simulink model "inverter_model"  (R2018b)
settings: Solver=VariableStepAuto  StartTime=0.0  StopTime=0.75  MaxStep=0.01  RelTol=1e-3  EnableMultiTasking=on
undefined symbols (not defined in the file): L, Lf, R, ron
libraries: powerlib x46, powerlib_meascontrol x11, simulink x9, peTransforms x5, simulink_extras x1
settings Model: Creator=vm-user  LastModifiedBy=suku (WPC)
settings DataIOCC: LimitDataPoints=on  SaveOutput=off  SaveTime=off
settings OptimizationCC: ExpressionDepthLimit=2147483647  LifeSpan=1
settings DebuggingCC: UnderspecifiedInitializationDetection=Classic  MergeDetectMultiDrivingBlocksExec=none  FcnCallInpInsideContextMsg=warning  AllowSymbolicDim=off  StateNameClashWarn=warning  LibraryContextMissingDiagnostic=none  SFUnexpectedBacktrackingDiag=warning  SFNoUnconditionalDefaultTransitionDiag=warning  SFExecutionAtInitializationDiag=none
settings SFSimCC: SimUseLocalCustomCode=off
settings RTWCC: RTWUseLocalCustomCode=off
settings CodeAppCC: StateflowObjectComments=on
settings GRTTargetCC: TargetLangStandard=C89/C90 (ANSI)  GeneratePreprocessorConditionals=Disable all  CombineOutputUpdateFcns=off  GRTInterface=on

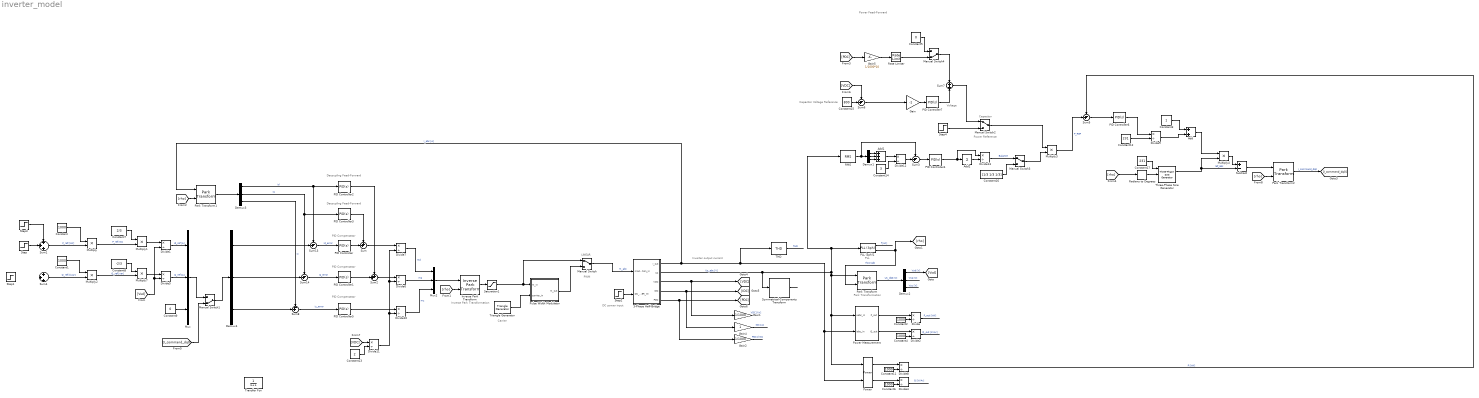
== system inverter_model ==
  note: Power Reference
  note: PLL
  note: PID Compensator
  note: PWM
  note: LINEAR
  note: Carrier
  note: Park Transformation
  note: Inverse Park Transformation
  note: Inverter output current
  note: Decoupling Feed-Forward
  note: Decoupling Feed-Forward
  note: Capacitor
  note: Capacitor Voltage Reference
  note: Power Feed-Forward
  note: Voltage
  note: DC power input
  note: PID Compensator
  note: PID Compensator
  3-Phase Half-Bridge : Subsystem
  Add : Sum
  Add1 : Sum  Inputs=+++
  Add2 : Sum  Inputs=+
  Constant{,1..2,4,6,11} (6 alike) : Constant  Value=1000
  Constant12 : Constant  Value=231
  Constant13 : Constant  Value=2
  Constant14 : Constant  Value=3
  Constant15 : Constant  Value=800
  Constant16 : Constant  Value=[1/3 1/3 1/3]
  Constant17 : Constant  Value=231
  Constant3 : Constant
  Constant5 : Constant  Value=0
  Constant7 : Constant  Value=2/3
  Constant8 : Constant  Value=-2/3
  Constant9 : Constant  Value=0
  Demux{1..4} (4 alike) : Demux  Outputs=3
  Divide{,1..2,4..13} (13 alike) : Product  Inputs=*/
  Gain : Gain  Gain=-1
  Gain1 : Gain  Gain=1/1000
  Gain2 : Gain  Gain=1/1000
  Gain4 : Gain
  Gain5 : Gain  Gain=1/1000*10
  Inverse Park Transform : peTransforms/Inverse Park Transform  AxisAlignment=Q-axis  PowerInvariant=off
  Manual Switch : ManualSwitch
  Manual Switch1 : ManualSwitch  CurrentSetting=0
  Manual Switch2 : ManualSwitch
  Manual Switch3 : ManualSwitch
  Manual Switch4 : ManualSwitch  CurrentSetting=0
  Multiply{,1..4,7} (6 alike) : Product
  Mux : Mux  Inputs=3
  Mux2 : Mux  Inputs=3
  PID Controller : simulink/Continuous/PID Controller  Controller=PID  Form=Parallel  TimeDomain=Continuous-time  SampleTime=-1  IntegratorMethod=Forward Euler  FilterMethod=Forward Euler  ControllerParametersSource=internal  P=1  I=100  D=0.25  UseFilter=on  N=100  TunerSelectOption=Transfer Function Based (PID Tuner App)  InitialConditionSource=internal  InitialConditionForIntegrator=0  InitialConditionForFilter=0  DifferentiatorICPrevScaledInput=0  ExternalReset=none  TrackingMode=off  Kt=1  LimitOutput=off  UpperSaturationLimit=inf  LowerSaturationLimit=-inf  LinearizeAsGain=on  AntiWindupMode=none  Kb=1  POutMin=[]  POutMax=[]  IOutMin=[]  IOutMax=[]  DOutMin=[]  DOutMax=[]  NOutMin=[]  NOutMax=[]  SumOutMin=[]  SumOutMax=[]  SaturationOutMin=[]  SaturationOutMax=[]  PParamMin=[]  PParamMax=[]  IParamMin=[]  IParamMax=[]  DParamMin=[]  DParamMax=[]  NParamMin=[]  NParamMax=[]  KbParamMin=[]  KbParamMax=[]  KtParamMin=[]  KtParamMax=[]  KbOutMin=[]  KbOutMax=[]  KtOutMin=[]  KtOutMax=[]  IntegratorOutMin=[]  IntegratorOutMax=[]  FilterOutMin=[]  FilterOutMax=[]  SumI1OutMin=[]  SumI1OutMax=[]  SumI2OutMin=[]  SumI2OutMax=[]  SumI3OutMin=[]  SumI3OutMax=[]  SumI4OutMin=[]  SumI4OutMax=[]  SumDOutMin=[]  SumDOutMax=[]  DifferentiatorOutMin=[]  DifferentiatorOutMax=[]  FilterDiffOutCoefMin=[]  FilterDiffOutCoefMax=[]  ReciprocalOutMin=[]  ReciprocalOutMax=[]  SumDenOutMin=[]  SumDenOutMax=[]  SumNumOutMin=[]  SumNumOutMax=[]  DivideOutMin=[]  DivideOutMax=[]  IntegratorContinuousStateAttributes=''  IntegratorStateMustResolveToSignalObject=off  IntegratorRTWStateStorageClass=Auto  FilterContinuousStateAttributes=''  FilterStateMustResolveToSignalObject=off  FilterRTWStateStorageClass=Auto  ParallelPVariant=InternalParameters  IdealPVariant=Disabled  IVariant=InternalParameters  DVariant=InternalParameters  IntegratorVariant=Continuous  SatVariant=Disabled  AWVariant=Passthrough  PCopyVariant=Disabled  TRVariant=Disabled  FdbkBlocksVariant=Forward  IdealPFdbkVariant=Disabled  SatFdbkVariant=Disabled  DerivativeFilterVariant=ContFilter  NVariant=InternalParameters  NCopyVariant=Disabled  FilterICVariant=InternalICsFilter  IntegratorICVariant=InternalICs  ExternalResetVariant=Disabled  TRSumVariant=Passthrough  SumFdbkVariant=Disabled  SumVariant=Sum_PID
  PID Controller1 : simulink/Continuous/PID Controller  Controller=PID  Form=Parallel  TimeDomain=Continuous-time  SampleTime=-1  IntegratorMethod=Forward Euler  FilterMethod=Forward Euler  ControllerParametersSource=internal  P=1  I=100  D=0.25  UseFilter=on  N=100  TunerSelectOption=Transfer Function Based (PID Tuner App)  InitialConditionSource=internal  InitialConditionForIntegrator=0  InitialConditionForFilter=0  DifferentiatorICPrevScaledInput=0  ExternalReset=none  TrackingMode=off  Kt=1  LimitOutput=off  UpperSaturationLimit=inf  LowerSaturationLimit=-inf  LinearizeAsGain=on  AntiWindupMode=none  Kb=1  POutMin=[]  POutMax=[]  IOutMin=[]  IOutMax=[]  DOutMin=[]  DOutMax=[]  NOutMin=[]  NOutMax=[]  SumOutMin=[]  SumOutMax=[]  SaturationOutMin=[]  SaturationOutMax=[]  PParamMin=[]  PParamMax=[]  IParamMin=[]  IParamMax=[]  DParamMin=[]  DParamMax=[]  NParamMin=[]  NParamMax=[]  KbParamMin=[]  KbParamMax=[]  KtParamMin=[]  KtParamMax=[]  KbOutMin=[]  KbOutMax=[]  KtOutMin=[]  KtOutMax=[]  IntegratorOutMin=[]  IntegratorOutMax=[]  FilterOutMin=[]  FilterOutMax=[]  SumI1OutMin=[]  SumI1OutMax=[]  SumI2OutMin=[]  SumI2OutMax=[]  SumI3OutMin=[]  SumI3OutMax=[]  SumI4OutMin=[]  SumI4OutMax=[]  SumDOutMin=[]  SumDOutMax=[]  DifferentiatorOutMin=[]  DifferentiatorOutMax=[]  FilterDiffOutCoefMin=[]  FilterDiffOutCoefMax=[]  ReciprocalOutMin=[]  ReciprocalOutMax=[]  SumDenOutMin=[]  SumDenOutMax=[]  SumNumOutMin=[]  SumNumOutMax=[]  DivideOutMin=[]  DivideOutMax=[]  IntegratorContinuousStateAttributes=''  IntegratorStateMustResolveToSignalObject=off  IntegratorRTWStateStorageClass=Auto  FilterContinuousStateAttributes=''  FilterStateMustResolveToSignalObject=off  FilterRTWStateStorageClass=Auto  ParallelPVariant=InternalParameters  IdealPVariant=Disabled  IVariant=InternalParameters  DVariant=InternalParameters  IntegratorVariant=Continuous  SatVariant=Disabled  AWVariant=Passthrough  PCopyVariant=Disabled  TRVariant=Disabled  FdbkBlocksVariant=Forward  IdealPFdbkVariant=Disabled  SatFdbkVariant=Disabled  DerivativeFilterVariant=ContFilter  NVariant=InternalParameters  NCopyVariant=Disabled  FilterICVariant=InternalICsFilter  IntegratorICVariant=InternalICs  ExternalResetVariant=Disabled  TRSumVariant=Passthrough  SumFdbkVariant=Disabled  SumVariant=Sum_PID
  PID Controller2 : simulink/Continuous/PID Controller  Controller=PID  Form=Parallel  TimeDomain=Continuous-time  SampleTime=-1  IntegratorMethod=Forward Euler  FilterMethod=Forward Euler  ControllerParametersSource=internal  P=0.22  I=0  D=0  UseFilter=on  N=100  TunerSelectOption=Transfer Function Based (PID Tuner App)  InitialConditionSource=internal  InitialConditionForIntegrator=0  InitialConditionForFilter=0  DifferentiatorICPrevScaledInput=0  ExternalReset=none  TrackingMode=off  Kt=1  LimitOutput=off  UpperSaturationLimit=inf  LowerSaturationLimit=-inf  LinearizeAsGain=on  AntiWindupMode=none  Kb=1  POutMin=[]  POutMax=[]  IOutMin=[]  IOutMax=[]  DOutMin=[]  DOutMax=[]  NOutMin=[]  NOutMax=[]  SumOutMin=[]  SumOutMax=[]  SaturationOutMin=[]  SaturationOutMax=[]  PParamMin=[]  PParamMax=[]  IParamMin=[]  IParamMax=[]  DParamMin=[]  DParamMax=[]  NParamMin=[]  NParamMax=[]  KbParamMin=[]  KbParamMax=[]  KtParamMin=[]  KtParamMax=[]  KbOutMin=[]  KbOutMax=[]  KtOutMin=[]  KtOutMax=[]  IntegratorOutMin=[]  IntegratorOutMax=[]  FilterOutMin=[]  FilterOutMax=[]  SumI1OutMin=[]  SumI1OutMax=[]  SumI2OutMin=[]  SumI2OutMax=[]  SumI3OutMin=[]  SumI3OutMax=[]  SumI4OutMin=[]  SumI4OutMax=[]  SumDOutMin=[]  SumDOutMax=[]  DifferentiatorOutMin=[]  DifferentiatorOutMax=[]  FilterDiffOutCoefMin=[]  FilterDiffOutCoefMax=[]  ReciprocalOutMin=[]  ReciprocalOutMax=[]  SumDenOutMin=[]  SumDenOutMax=[]  SumNumOutMin=[]  SumNumOutMax=[]  DivideOutMin=[]  DivideOutMax=[]  IntegratorContinuousStateAttributes=''  IntegratorStateMustResolveToSignalObject=off  IntegratorRTWStateStorageClass=Auto  FilterContinuousStateAttributes=''  FilterStateMustResolveToSignalObject=off  FilterRTWStateStorageClass=Auto  ParallelPVariant=InternalParameters  IdealPVariant=Disabled  IVariant=InternalParameters  DVariant=InternalParameters  IntegratorVariant=Continuous  SatVariant=Disabled  AWVariant=Passthrough  PCopyVariant=Disabled  TRVariant=Disabled  FdbkBlocksVariant=Forward  IdealPFdbkVariant=Disabled  SatFdbkVariant=Disabled  DerivativeFilterVariant=ContFilter  NVariant=InternalParameters  NCopyVariant=Disabled  FilterICVariant=InternalICsFilter  IntegratorICVariant=InternalICs  ExternalResetVariant=Disabled  TRSumVariant=Passthrough  SumFdbkVariant=Disabled  SumVariant=Sum_PID
  PID Controller3 : simulink/Continuous/PID Controller  Controller=PID  Form=Parallel  TimeDomain=Continuous-time  SampleTime=-1  IntegratorMethod=Forward Euler  FilterMethod=Forward Euler  ControllerParametersSource=internal  P=-0.22  I=0  D=0  UseFilter=on  N=100  TunerSelectOption=Transfer Function Based (PID Tuner App)  InitialConditionSource=internal  InitialConditionForIntegrator=0  InitialConditionForFilter=0  DifferentiatorICPrevScaledInput=0  ExternalReset=none  TrackingMode=off  Kt=1  LimitOutput=off  UpperSaturationLimit=inf  LowerSaturationLimit=-inf  LinearizeAsGain=on  AntiWindupMode=none  Kb=1  POutMin=[]  POutMax=[]  IOutMin=[]  IOutMax=[]  DOutMin=[]  DOutMax=[]  NOutMin=[]  NOutMax=[]  SumOutMin=[]  SumOutMax=[]  SaturationOutMin=[]  SaturationOutMax=[]  PParamMin=[]  PParamMax=[]  IParamMin=[]  IParamMax=[]  DParamMin=[]  DParamMax=[]  NParamMin=[]  NParamMax=[]  KbParamMin=[]  KbParamMax=[]  KtParamMin=[]  KtParamMax=[]  KbOutMin=[]  KbOutMax=[]  KtOutMin=[]  KtOutMax=[]  IntegratorOutMin=[]  IntegratorOutMax=[]  FilterOutMin=[]  FilterOutMax=[]  SumI1OutMin=[]  SumI1OutMax=[]  SumI2OutMin=[]  SumI2OutMax=[]  SumI3OutMin=[]  SumI3OutMax=[]  SumI4OutMin=[]  SumI4OutMax=[]  SumDOutMin=[]  SumDOutMax=[]  DifferentiatorOutMin=[]  DifferentiatorOutMax=[]  FilterDiffOutCoefMin=[]  FilterDiffOutCoefMax=[]  ReciprocalOutMin=[]  ReciprocalOutMax=[]  SumDenOutMin=[]  SumDenOutMax=[]  SumNumOutMin=[]  SumNumOutMax=[]  DivideOutMin=[]  DivideOutMax=[]  IntegratorContinuousStateAttributes=''  IntegratorStateMustResolveToSignalObject=off  IntegratorRTWStateStorageClass=Auto  FilterContinuousStateAttributes=''  FilterStateMustResolveToSignalObject=off  FilterRTWStateStorageClass=Auto  ParallelPVariant=InternalParameters  IdealPVariant=Disabled  IVariant=InternalParameters  DVariant=InternalParameters  IntegratorVariant=Continuous  SatVariant=Disabled  AWVariant=Passthrough  PCopyVariant=Disabled  TRVariant=Disabled  FdbkBlocksVariant=Forward  IdealPFdbkVariant=Disabled  SatFdbkVariant=Disabled  DerivativeFilterVariant=ContFilter  NVariant=InternalParameters  NCopyVariant=Disabled  FilterICVariant=InternalICsFilter  IntegratorICVariant=InternalICs  ExternalResetVariant=Disabled  TRSumVariant=Passthrough  SumFdbkVariant=Disabled  SumVariant=Sum_PID
  PID Controller4 : simulink/Continuous/PID Controller  Controller=PID  Form=Parallel  TimeDomain=Continuous-time  SampleTime=-1  IntegratorMethod=Forward Euler  FilterMethod=Forward Euler  ControllerParametersSource=internal  P=0.1  I=1  D=0  UseFilter=on  N=100  TunerSelectOption=Transfer Function Based (PID Tuner App)  InitialConditionSource=internal  InitialConditionForIntegrator=1/3  InitialConditionForFilter=0  DifferentiatorICPrevScaledInput=0  ExternalReset=none  TrackingMode=off  Kt=1  LimitOutput=on  UpperSaturationLimit=0.9  LowerSaturationLimit=0.1  LinearizeAsGain=on  AntiWindupMode=clamping  Kb=1  POutMin=[]  POutMax=[]  IOutMin=[]  IOutMax=[]  DOutMin=[]  DOutMax=[]  NOutMin=[]  NOutMax=[]  SumOutMin=[]  SumOutMax=[]  SaturationOutMin=[]  SaturationOutMax=[]  PParamMin=[]  PParamMax=[]  IParamMin=[]  IParamMax=[]  DParamMin=[]  DParamMax=[]  NParamMin=[]  NParamMax=[]  KbParamMin=[]  KbParamMax=[]  KtParamMin=[]  KtParamMax=[]  KbOutMin=[]  KbOutMax=[]  KtOutMin=[]  KtOutMax=[]  IntegratorOutMin=[]  IntegratorOutMax=[]  FilterOutMin=[]  FilterOutMax=[]  SumI1OutMin=[]  SumI1OutMax=[]  SumI2OutMin=[]  SumI2OutMax=[]  SumI3OutMin=[]  SumI3OutMax=[]  SumI4OutMin=[]  SumI4OutMax=[]  SumDOutMin=[]  SumDOutMax=[]  DifferentiatorOutMin=[]  DifferentiatorOutMax=[]  FilterDiffOutCoefMin=[]  FilterDiffOutCoefMax=[]  ReciprocalOutMin=[]  ReciprocalOutMax=[]  SumDenOutMin=[]  SumDenOutMax=[]  SumNumOutMin=[]  SumNumOutMax=[]  DivideOutMin=[]  DivideOutMax=[]  IntegratorContinuousStateAttributes=''  IntegratorStateMustResolveToSignalObject=off  IntegratorRTWStateStorageClass=Auto  FilterContinuousStateAttributes=''  FilterStateMustResolveToSignalObject=off  FilterRTWStateStorageClass=Auto  ParallelPVariant=InternalParameters  IdealPVariant=Disabled  IVariant=InternalParameters  DVariant=InternalParameters  IntegratorVariant=Continuous  SatVariant=Enabled  AWVariant=ContClampingParallel  PCopyVariant=Disabled  TRVariant=Disabled  FdbkBlocksVariant=Forward  IdealPFdbkVariant=Disabled  SatFdbkVariant=Disabled  DerivativeFilterVariant=ContFilter  NVariant=InternalParameters  NCopyVariant=Disabled  FilterICVariant=InternalICsFilter  IntegratorICVariant=InternalICs  ExternalResetVariant=Disabled  TRSumVariant=Passthrough  SumFdbkVariant=Disabled  SumVariant=Sum_PID
  PID Controller5 : simulink/Continuous/PID Controller  Controller=PID  Form=Parallel  TimeDomain=Continuous-time  SampleTime=-1  IntegratorMethod=Forward Euler  FilterMethod=Forward Euler  ControllerParametersSource=internal  P=1  I=100  D=0.25  UseFilter=on  N=100  TunerSelectOption=Transfer Function Based (PID Tuner App)  InitialConditionSource=internal  InitialConditionForIntegrator=0  InitialConditionForFilter=0  DifferentiatorICPrevScaledInput=0  ExternalReset=none  TrackingMode=off  Kt=1  LimitOutput=off  UpperSaturationLimit=inf  LowerSaturationLimit=-inf  LinearizeAsGain=on  AntiWindupMode=none  Kb=1  POutMin=[]  POutMax=[]  IOutMin=[]  IOutMax=[]  DOutMin=[]  DOutMax=[]  NOutMin=[]  NOutMax=[]  SumOutMin=[]  SumOutMax=[]  SaturationOutMin=[]  SaturationOutMax=[]  PParamMin=[]  PParamMax=[]  IParamMin=[]  IParamMax=[]  DParamMin=[]  DParamMax=[]  NParamMin=[]  NParamMax=[]  KbParamMin=[]  KbParamMax=[]  KtParamMin=[]  KtParamMax=[]  KbOutMin=[]  KbOutMax=[]  KtOutMin=[]  KtOutMax=[]  IntegratorOutMin=[]  IntegratorOutMax=[]  FilterOutMin=[]  FilterOutMax=[]  SumI1OutMin=[]  SumI1OutMax=[]  SumI2OutMin=[]  SumI2OutMax=[]  SumI3OutMin=[]  SumI3OutMax=[]  SumI4OutMin=[]  SumI4OutMax=[]  SumDOutMin=[]  SumDOutMax=[]  DifferentiatorOutMin=[]  DifferentiatorOutMax=[]  FilterDiffOutCoefMin=[]  FilterDiffOutCoefMax=[]  ReciprocalOutMin=[]  ReciprocalOutMax=[]  SumDenOutMin=[]  SumDenOutMax=[]  SumNumOutMin=[]  SumNumOutMax=[]  DivideOutMin=[]  DivideOutMax=[]  IntegratorContinuousStateAttributes=''  IntegratorStateMustResolveToSignalObject=off  IntegratorRTWStateStorageClass=Auto  FilterContinuousStateAttributes=''  FilterStateMustResolveToSignalObject=off  FilterRTWStateStorageClass=Auto  ParallelPVariant=InternalParameters  IdealPVariant=Disabled  IVariant=InternalParameters  DVariant=InternalParameters  IntegratorVariant=Continuous  SatVariant=Disabled  AWVariant=Passthrough  PCopyVariant=Disabled  TRVariant=Disabled  FdbkBlocksVariant=Forward  IdealPFdbkVariant=Disabled  SatFdbkVariant=Disabled  DerivativeFilterVariant=ContFilter  NVariant=InternalParameters  NCopyVariant=Disabled  FilterICVariant=InternalICsFilter  IntegratorICVariant=InternalICs  ExternalResetVariant=Disabled  TRSumVariant=Passthrough  SumFdbkVariant=Disabled  SumVariant=Sum_PID
  PID Controller6 : simulink/Continuous/PID Controller  Controller=PID  Form=Parallel  TimeDomain=Continuous-time  SampleTime=-1  IntegratorMethod=Forward Euler  FilterMethod=Forward Euler  ControllerParametersSource=internal  P=1  I=1  D=0  UseFilter=on  N=100  TunerSelectOption=Transfer Function Based (PID Tuner App)  InitialConditionSource=internal  InitialConditionForIntegrator=0  InitialConditionForFilter=0  DifferentiatorICPrevScaledInput=0  ExternalReset=none  TrackingMode=off  Kt=1  LimitOutput=on  UpperSaturationLimit=100  LowerSaturationLimit=0  LinearizeAsGain=on  AntiWindupMode=none  Kb=1  POutMin=[]  POutMax=[]  IOutMin=[]  IOutMax=[]  DOutMin=[]  DOutMax=[]  NOutMin=[]  NOutMax=[]  SumOutMin=[]  SumOutMax=[]  SaturationOutMin=[]  SaturationOutMax=[]  PParamMin=[]  PParamMax=[]  IParamMin=[]  IParamMax=[]  DParamMin=[]  DParamMax=[]  NParamMin=[]  NParamMax=[]  KbParamMin=[]  KbParamMax=[]  KtParamMin=[]  KtParamMax=[]  KbOutMin=[]  KbOutMax=[]  KtOutMin=[]  KtOutMax=[]  IntegratorOutMin=[]  IntegratorOutMax=[]  FilterOutMin=[]  FilterOutMax=[]  SumI1OutMin=[]  SumI1OutMax=[]  SumI2OutMin=[]  SumI2OutMax=[]  SumI3OutMin=[]  SumI3OutMax=[]  SumI4OutMin=[]  SumI4OutMax=[]  SumDOutMin=[]  SumDOutMax=[]  DifferentiatorOutMin=[]  DifferentiatorOutMax=[]  FilterDiffOutCoefMin=[]  FilterDiffOutCoefMax=[]  ReciprocalOutMin=[]  ReciprocalOutMax=[]  SumDenOutMin=[]  SumDenOutMax=[]  SumNumOutMin=[]  SumNumOutMax=[]  DivideOutMin=[]  DivideOutMax=[]  IntegratorContinuousStateAttributes=''  IntegratorStateMustResolveToSignalObject=off  IntegratorRTWStateStorageClass=Auto  FilterContinuousStateAttributes=''  FilterStateMustResolveToSignalObject=off  FilterRTWStateStorageClass=Auto  ParallelPVariant=InternalParameters  IdealPVariant=Disabled  IVariant=InternalParameters  DVariant=InternalParameters  IntegratorVariant=Continuous  SatVariant=Enabled  AWVariant=Passthrough  PCopyVariant=Disabled  TRVariant=Disabled  FdbkBlocksVariant=Forward  IdealPFdbkVariant=Disabled  SatFdbkVariant=Disabled  DerivativeFilterVariant=ContFilter  NVariant=InternalParameters  NCopyVariant=Disabled  FilterICVariant=InternalICsFilter  IntegratorICVariant=InternalICs  ExternalResetVariant=Disabled  TRSumVariant=Passthrough  SumFdbkVariant=Disabled  SumVariant=Sum_PID
  PID Controller7 : simulink/Continuous/PID Controller  Controller=PID  Form=Parallel  TimeDomain=Continuous-time  SampleTime=-1  IntegratorMethod=Forward Euler  FilterMethod=Forward Euler  ControllerParametersSource=internal  P=1.5  I=0.5  D=0  UseFilter=on  N=100  TunerSelectOption=Transfer Function Based (PID Tuner App)  InitialConditionSource=internal  InitialConditionForIntegrator=0  InitialConditionForFilter=0  DifferentiatorICPrevScaledInput=0  ExternalReset=none  TrackingMode=off  Kt=1  LimitOutput=off  UpperSaturationLimit=100  LowerSaturationLimit=100  LinearizeAsGain=off  AntiWindupMode=clamping  Kb=1  POutMin=[]  POutMax=[]  IOutMin=[]  IOutMax=[]  DOutMin=[]  DOutMax=[]  NOutMin=[]  NOutMax=[]  SumOutMin=[]  SumOutMax=[]  SaturationOutMin=[]  SaturationOutMax=[]  PParamMin=[]  PParamMax=[]  IParamMin=[]  IParamMax=[]  DParamMin=[]  DParamMax=[]  NParamMin=[]  NParamMax=[]  KbParamMin=[]  KbParamMax=[]  KtParamMin=[]  KtParamMax=[]  KbOutMin=[]  KbOutMax=[]  KtOutMin=[]  KtOutMax=[]  IntegratorOutMin=[]  IntegratorOutMax=[]  FilterOutMin=[]  FilterOutMax=[]  SumI1OutMin=[]  SumI1OutMax=[]  SumI2OutMin=[]  SumI2OutMax=[]  SumI3OutMin=[]  SumI3OutMax=[]  SumI4OutMin=[]  SumI4OutMax=[]  SumDOutMin=[]  SumDOutMax=[]  DifferentiatorOutMin=[]  DifferentiatorOutMax=[]  FilterDiffOutCoefMin=[]  FilterDiffOutCoefMax=[]  ReciprocalOutMin=[]  ReciprocalOutMax=[]  SumDenOutMin=[]  SumDenOutMax=[]  SumNumOutMin=[]  SumNumOutMax=[]  DivideOutMin=[]  DivideOutMax=[]  IntegratorContinuousStateAttributes=''  IntegratorStateMustResolveToSignalObject=off  IntegratorRTWStateStorageClass=Auto  FilterContinuousStateAttributes=''  FilterStateMustResolveToSignalObject=off  FilterRTWStateStorageClass=Auto  ParallelPVariant=InternalParameters  IdealPVariant=Disabled  IVariant=InternalParameters  DVariant=InternalParameters  IntegratorVariant=Continuous  SatVariant=Disabled  AWVariant=Passthrough  PCopyVariant=Disabled  TRVariant=Disabled  FdbkBlocksVariant=Forward  IdealPFdbkVariant=Disabled  SatFdbkVariant=Disabled  DerivativeFilterVariant=ContFilter  NVariant=InternalParameters  NCopyVariant=Disabled  FilterICVariant=InternalICsFilter  IntegratorICVariant=InternalICs  ExternalResetVariant=Disabled  TRSumVariant=Passthrough  SumFdbkVariant=Disabled  SumVariant=Sum_PID
  PLL (3ph)1 : powerlib_meascontrol/PLL/PLL (3ph)  Fmin=40  Par_Init=[0, 50]  ParK=[180, 3200, 1]  TcD=1e-4  MaxRateChangeFreq=12  FilterCutOffFreq=25  Ts=0  AGC=on
      settings: SourceProductName=Simscape Electrical
  Park Transform : peTransforms/Park Transform  AxisAlignment=Q-axis  PowerInvariant=off
  Park Transform1 : peTransforms/Park Transform  AxisAlignment=Q-axis  PowerInvariant=off
  Park Transform2 : peTransforms/Park Transform  AxisAlignment=Q-axis  PowerInvariant=off
  Power : powerlib_meascontrol/Measurements/Power  Freq=50  Vinit=[1, 0]  Iinit=[1, 0]  Ts=0
      settings: SourceProductName=Simscape Electrical
  Power Measurement : Subsystem
  Pulse Width Modulator : Subsystem
  RMS : powerlib_meascontrol/Measurements/RMS  TrueRMS=on  Freq=50  RMSInit=231  Ts=0
  Radians to Degrees : simulink_extras/Transformations/Radians to Degrees
  Rate Limiter : RateLimiter  RisingSlewLimit=1000  FallingSlewLimit=-1000  SampleTimeMode=inherited
  Saturation1 : Saturate  UpperLimit=1  LowerLimit=-1
  Step : Step  Time=0.05  After=8  SampleTime=0
  Step1 : Step  Time=0.5  After=6  SampleTime=0
  Step2 : Step  Time=0.05  After=10000  SampleTime=0
  Step3 : Step  Time=0.5  After=-4  SampleTime=0
  Step4 : Step  Time=0.05  After=10000  SampleTime=0
  Subtract : Sum  Inputs=+-
  Sum : Sum  Inputs=++|
  Sum1 : Sum  Inputs=+|+|+
  Sum{3,5..6,8,13..14} (6 alike) : Sum  Inputs=-+|
  Sum2 : Sum  Inputs=++|
  Sum4 : Sum  Inputs=+|+|+
  Sum7 : Sum
  Symmetrical-Components Transform : peTransforms/Symmetrical-Components Transform  PowerInvariant=off
  THD : powerlib_meascontrol/Measurements/THD  Freq=50  Ts=0
      settings: SourceProductName=Simscape Electrical
  Three-Phase Sine Generator : powerlib_meascontrol/Pulse & Signal Generators/Three-Phase Sine Generator  Ts=0
      settings: SourceProductName=Simscape Power Systems  SourceProductBaseCode=PS
  Transfer Fcn : TransferFcn  Denominator=[1 1]
  Triangle Generator : powerlib_meascontrol/Pulse & Signal Generators/Triangle Generator  Freq=1e3  Phase=0  Ts=0
      settings: SourceProductName=Simscape Electrical
  wires:
  3-Phase Half-Bridge/2(Us) -> Power/1, Power Measurement/1(uabc_in), Park Transform/1, RMS/1, PLL (3ph)1/1, Symmetrical-Components Transform/1  "Us_abc [V]"
  PLL (3ph)1/2 -> Park Transform/2, [rho]  "rho [rad]"
  Park Transform/1 -> Demux2/1  "Us_dq0 [V]"
  Demux2/1 -> [Vsd]  "Vsd [V]"
  Demux2/3 -> ?  "Vsz [V]"
  Park Transform1/1 -> Demux3/1
  Demux3/3 -> Sum8/1  "iz"
  Sum1/1 -> Multiply/2  "P_ref [kW]"
  Sum4/1 -> Multiply2/2  "Q_ref [kvar]"
  Constant7/1 -> Multiply1/1
  Constant8/1 -> Multiply7/1
  Multiply1/1 -> Divide1/1
  Multiply7/1 -> Divide5/1
  Divide1/1 -> Mux/1  "id_ref [A]"
  Divide5/1 -> Mux/2  "iq_ref [A]"
  Sum13/1 -> PID Controller/1  "id_error"
  PID Controller/1 -> Sum/2
  Sum14/1 -> PID Controller1/1  "iq_error"
  Mux2/1 -> Inverse Park Transform/1
  Divide11/1 -> Divide10/2, Divide7/2, Divide6/2
  Divide7/1 -> Mux2/1  "md"
  Divide6/1 -> Mux2/2  "mq"
  Inverse Park Transform/1 -> Saturation1/1
  Demux3/2 -> Sum14/1, PID Controller3/1  "iq"
  Demux3/1 -> Sum13/1, PID Controller2/1  "id"
  Triangle Generator/1 -> Pulse Width Modulator/2(carrier_in)
  Pulse Width Modulator/1("m_out ") -> Manual Switch/2
  3-Phase Half-Bridge/1(i_out) -> THD/1, Power/2, Power Measurement/2(iabc_in), Park Transform1/1  "i_abc [A]"
  Manual Switch/1 -> 3-Phase Half-Bridge/1(modulation_in)  "m_abc"
  Constant/1 -> Multiply/1
  Multiply/1 -> Multiply1/2  "P_ref [W]"
  Constant1/1 -> Multiply2/1
  Multiply2/1 -> Multiply7/2  "Q_ref [var]"
  Constant2/1 -> Divide/2
  Divide2/1 -> ?  "Q_out [kVAr]"
  Power Measurement/1(P_out) -> Divide/1
  Power Measurement/2(Q_out) -> Divide2/1
  Constant4/1 -> Divide2/2
  Demux2/2 -> ?  "Vsq [V]"
  [Vsd] -> Divide1/2, Divide5/2
  [rho] -> Inverse Park Transform/2
  [rho] -> Park Transform1/2
  Step/1 -> Sum1/2
  THD/1 -> ?  "THD"
  Sum/1 -> Divide7/1
  Sum2/1 -> Divide6/1
  PID Controller1/1 -> Sum2/2
  PID Controller2/1 -> Sum2/1
  PID Controller3/1 -> Sum/1
  Power/1 -> Divide8/1
  Divide4/1 -> ?  "Q [kVAr]"
  Constant6/1 -> Divide4/2
  Constant11/1 -> Divide8/2
  Power/2 -> Divide4/1
  Saturation1/1 -> Manual Switch/1, Pulse Width Modulator/1(m_in)
  Step3/1 -> Sum1/1
  Park Transform2/1 -> [I_command_dq0]  "I_command_dq0"
  PID Controller5/1 -> Divide10/1
  Sum8/1 -> PID Controller5/1  "iz_error"
  Demux4/2 -> Sum14/2
  Demux4/3 -> Sum8/2
  Demux4/1 -> Sum13/2
  Sum5/1 -> PID Controller6/1
  Multiply4/1 -> Subtract/1
  Divide8/1 -> Sum5/1  "P [kW]"
  Constant3/1 -> Add/1
  Divide9/1 -> Add/2
  Add/1 -> Multiply4/1
  RMS/1 -> Sum3/1, Demux1/1
  Constant12/1 -> Divide9/2
  Subtract/1 -> Park Transform2/1
  Divide/1 -> ?  "P_out [kW]"
  Demux1/1 -> Add1/1
  Demux1/2 -> Add1/2
  Demux1/3 -> Add1/3
  Add1/1 -> Divide12/1
  Constant14/1 -> Divide12/2
  Divide12/1 -> Sum3/2
  Sum3/1 -> PID Controller4/1
  PID Controller4/1 -> Divide13/1, Add2/1
  Add2/1 -> Divide13/2
  Divide13/1 -> Manual Switch3/1  "Balance"
  Manual Switch2/1 -> Multiply3/1
  Multiply3/1 -> Sum5/2  "P_REF"
  Constant13/1 -> Divide11/2
  3-Phase Half-Bridge/3(VDC) -> Gain1/1, [VDC]
  Constant9/1 -> Mux/3
  Manual Switch1/1 -> Demux4/1
  Mux/1 -> Manual Switch1/1
  [I_command_dq0] -> Manual Switch1/2
  Divide10/1 -> Mux2/3  "mz"
  Step4/1 -> Manual Switch2/2
  Manual Switch3/1 -> Multiply3/2
  Constant16/1 -> Manual Switch3/2
  Radians to Degrees/1 -> Three-Phase Sine Generator/2
  Three-Phase Sine Generator/1 -> Multiply4/2, Subtract/2  "ref_abc"
  [rho] -> Radians to Degrees/1
  Constant17/1 -> Three-Phase Sine Generator/1
  PLL (3ph)1/1 -> ?  "f [Hz]"
  Constant15/1 -> Sum6/2
  Gain/1 -> PID Controller7/1
  [VDC] -> Sum6/1
  Gain1/1 -> ?  "VDC [kV]"
  [VDC] -> Divide11/1
  3-Phase Half-Bridge/4(IDC) -> Gain4/1, [IDC]
  Gain2/1 -> ?  "PDC [kW]"
  PID Controller7/1 -> Sum7/2
  Manual Switch4/1 -> Sum7/1
  Sum7/1 -> Manual Switch2/1
  3-Phase Half-Bridge/5(PDC) -> [PDC], Gain2/1
  Gain4/1 -> ?  "IDC [A]"
  Rate Limiter/1 -> Manual Switch4/2
  Constant5/1 -> Manual Switch4/1
  [PDC] -> Gain5/1
  Gain5/1 -> Rate Limiter/1
  Sum6/1 -> Gain/1
  Symmetrical-Components Transform/1 -> ?
  Step2/1 -> 3-Phase Half-Bridge/2(DC_POWER_IN)
  [rho] -> Park Transform2/2
  PID Controller6/1 -> Divide9/1

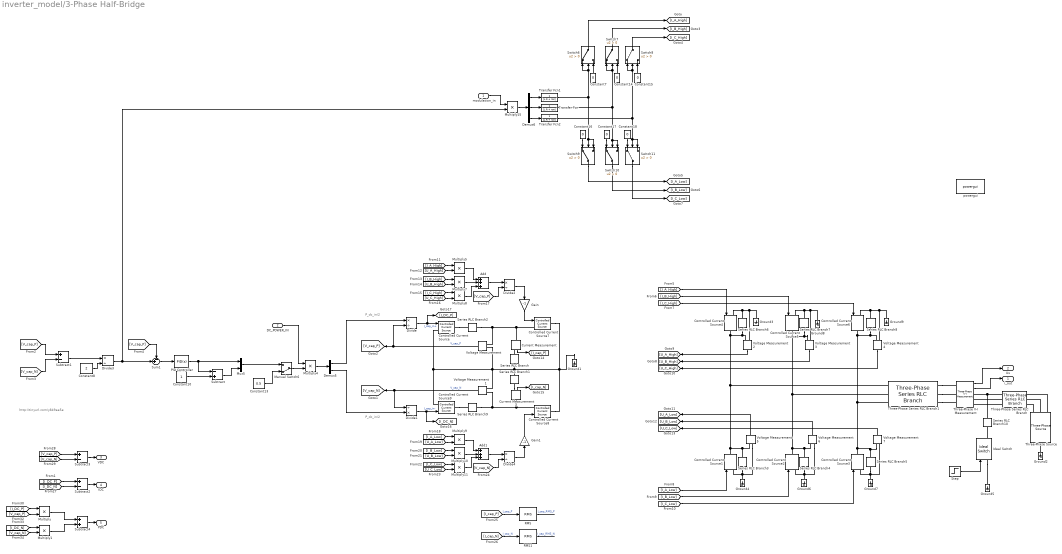
== system inverter_model/3-Phase Half-Bridge ==
  note: P_dc_in/2
  note: http://tinyurl.com/y849ae5e
  note: P_dc_in/2
  modulation_in : Inport
  DC_POWER_IN : Inport  Port=2
  Add : Sum  Inputs=3
  Add1 : Sum  Inputs=3
  Constant10 : Constant
  Constant13 : Constant  Value=0.5
  Constant{7,14..18} (6 alike) : Constant  Value=0
  Constant8 : Constant  Value=2
  Controlled Current Source{,1..9} (10 alike) : powerlib/Electrical Sources/Controlled Current Source  Initialize=on  Source_Type=DC  Amplitude=0  Phase=0  Frequency=0  Measurements=None
  Current Measurement : powerlib/Measurements/Current Measurement  PhasorSimulation=off  OutputType=Complex  PSBequivalent=0
  Current Measurement1 : powerlib/Measurements/Current Measurement  PhasorSimulation=off  OutputType=Complex  PSBequivalent=0
  Demux5 : Demux  Outputs=2
  Demux6 : Demux  Outputs=3
  Divide{,2..4} (4 alike) : Product  Inputs=*/
  Divide1 : Product  Inputs=/*
  Gain : Gain  Gain=-1
  Gain1 : Gain  Gain=-1
  Ground{1..9} (9 alike) : powerlib/Elements/Ground  LConnTagsString=a
      settings: SourceProductName=Simscape Electrical
  Ideal Switch : powerlib/Power Electronics/Ideal Switch  Ron=0.001  Lon=0  IC=0  Rs=1e5  Cs=inf  Measurements=on
  Manual Switch6 : ManualSwitch  CurrentSetting=0
  Multiply{,1,4..5,7..11,15} (10 alike) : Product
  Mux5 : Mux  Inputs=2
  PID Controller : simulink/Continuous/PID Controller  Controller=PID  Form=Parallel  TimeDomain=Continuous-time  SampleTime=-1  IntegratorMethod=Forward Euler  FilterMethod=Forward Euler  ControllerParametersSource=internal  P=1  I=1  D=0  UseFilter=on  N=100  TunerSelectOption=Transfer Function Based (PID Tuner App)  InitialConditionSource=internal  InitialConditionForIntegrator=0.5  InitialConditionForFilter=0  DifferentiatorICPrevScaledInput=0  ExternalReset=none  TrackingMode=off  Kt=1  LimitOutput=on  UpperSaturationLimit=inf  LowerSaturationLimit=0.1  LinearizeAsGain=on  AntiWindupMode=none  Kb=1  POutMin=[]  POutMax=[]  IOutMin=[]  IOutMax=[]  DOutMin=[]  DOutMax=[]  NOutMin=[]  NOutMax=[]  SumOutMin=[]  SumOutMax=[]  SaturationOutMin=[]  SaturationOutMax=[]  PParamMin=[]  PParamMax=[]  IParamMin=[]  IParamMax=[]  DParamMin=[]  DParamMax=[]  NParamMin=[]  NParamMax=[]  KbParamMin=[]  KbParamMax=[]  KtParamMin=[]  KtParamMax=[]  KbOutMin=[]  KbOutMax=[]  KtOutMin=[]  KtOutMax=[]  IntegratorOutMin=[]  IntegratorOutMax=[]  FilterOutMin=[]  FilterOutMax=[]  SumI1OutMin=[]  SumI1OutMax=[]  SumI2OutMin=[]  SumI2OutMax=[]  SumI3OutMin=[]  SumI3OutMax=[]  SumI4OutMin=[]  SumI4OutMax=[]  SumDOutMin=[]  SumDOutMax=[]  DifferentiatorOutMin=[]  DifferentiatorOutMax=[]  FilterDiffOutCoefMin=[]  FilterDiffOutCoefMax=[]  ReciprocalOutMin=[]  ReciprocalOutMax=[]  SumDenOutMin=[]  SumDenOutMax=[]  SumNumOutMin=[]  SumNumOutMax=[]  DivideOutMin=[]  DivideOutMax=[]  IntegratorContinuousStateAttributes=''  IntegratorStateMustResolveToSignalObject=off  IntegratorRTWStateStorageClass=Auto  FilterContinuousStateAttributes=''  FilterStateMustResolveToSignalObject=off  FilterRTWStateStorageClass=Auto  ParallelPVariant=InternalParameters  IdealPVariant=Disabled  IVariant=InternalParameters  DVariant=InternalParameters  IntegratorVariant=Continuous  SatVariant=Enabled  AWVariant=Passthrough  PCopyVariant=Disabled  TRVariant=Disabled  FdbkBlocksVariant=Forward  IdealPFdbkVariant=Disabled  SatFdbkVariant=Disabled  DerivativeFilterVariant=ContFilter  NVariant=InternalParameters  NCopyVariant=Disabled  FilterICVariant=InternalICsFilter  IntegratorICVariant=InternalICs  ExternalResetVariant=Disabled  TRSumVariant=Passthrough  SumFdbkVariant=Disabled  SumVariant=Sum_PID
  RMS : powerlib_meascontrol/Measurements/RMS  TrueRMS=on  Freq=50  RMSInit=120  Ts=0
  RMS1 : powerlib_meascontrol/Measurements/RMS  TrueRMS=on  Freq=50  RMSInit=120  Ts=0
  Series RLC Branch : powerlib/Elements/Series RLC Branch  LConnTagsString=__new0  RConnTagsString=__new0  BranchType=C  Resistance=1  Inductance=1e-3  SetiL0=off  InitialCurrent=0  Capacitance=470e-6  Setx0=on  InitialVoltage=100  Measurements=None
  Series RLC Branch1 : powerlib/Elements/Series RLC Branch  LConnTagsString=__new0  RConnTagsString=__new0  BranchType=C  Resistance=1  Inductance=1e-3  SetiL0=off  InitialCurrent=0  Capacitance=470e-6  Setx0=on  InitialVoltage=100  Measurements=None
  Series RLC Branch10 : powerlib/Elements/Series RLC Branch  LConnTagsString=__new0  RConnTagsString=__new0  BranchType=R  Resistance=10  Inductance=1e-3  SetiL0=off  InitialCurrent=0  Capacitance=47000e-6  Setx0=on  InitialVoltage=300  Measurements=None
  Series RLC Branch2 : powerlib/Elements/Series RLC Branch  LConnTagsString=__new0  RConnTagsString=__new0  BranchType=R  Resistance=1  Inductance=1e-3  SetiL0=off  InitialCurrent=0  Capacitance=470e-6  Setx0=on  InitialVoltage=300  Measurements=None
  Series RLC Branch{3..8} (6 alike) : powerlib/Elements/Series RLC Branch  LConnTagsString=__new0  RConnTagsString=__new0  BranchType=R  Resistance=5000  Inductance=1e-3  SetiL0=off  InitialCurrent=0  Capacitance=47000e-6  Setx0=on  InitialVoltage=300  Measurements=None
  Series RLC Branch9 : powerlib/Elements/Series RLC Branch  LConnTagsString=__new0  RConnTagsString=__new0  BranchType=R  Resistance=1  Inductance=1e-3  SetiL0=off  InitialCurrent=0  Capacitance=470e-6  Setx0=on  InitialVoltage=300  Measurements=None
  Step : Step  Time=0.25  SampleTime=0
  Subtract : Sum  Inputs=-+
  Subtract1 : Sum  Inputs=+-
  Subtract2 : Sum  Inputs=+-
  Subtract3 : Sum  Inputs=+-
  Subtract4 : Sum
  Sum1 : Sum  Inputs=-+|
  Switch{6..11} (6 alike) : Switch  Criteria=u2 > Threshold
  Three-Phase Series RLC Branch : powerlib/Elements/Three-Phase Series RLC Branch  LConnTagsString=A|B|C  RConnTagsString=A|B|C  BranchType=RL  Resistance=1  Inductance=Lf  Capacitance=1e-6  Measurements=None
  Three-Phase Series RLC Branch1 : powerlib/Elements/Three-Phase Series RLC Branch  LConnTagsString=A|B|C  RConnTagsString=A|B|C  BranchType=RL  Resistance=R + ron  Inductance=L  Capacitance=1e-6  Measurements=None
  Three-Phase V-I Measurement : powerlib/Measurements/Three-Phase V-I Measurement  VoltageMeasurement=phase-to-ground  SetLabelV=off  LabelV=Vabc  Vpu=off  VpuLL=off  CurrentMeasurement=yes  SetLabelI=off  LabelI=Iabc  Ipu=off  Pbase=100e6  Vbase=500e3  OutputType=Complex  PhasorSimulation=off  PSBequivalent=0
  Three-Phase Source : powerlib/Electrical Sources/Three-Phase Source  InternalConnection=Yn  VoltagePhases=off  Voltage=400  PhaseAngle=0  Voltage_phases=[25e3 25e3 25e3]/sqrt(3)  PhaseAngles_phases=[0 -120 +120]  Frequency=50  NonIdealSource=off  SpecifyImpedance=off  Resistance=0.8929  Inductance=16.58e-3  ShortCircuitLevel=100e6  BaseVoltage=25e3  XRratio=7  BusType=swing  Pref=10e3  Qref=0  Prefabc=[10e3, 10e3, 10e3]  Qrefabc=[0, 0, 0]  Qmin=-inf  Qmax=inf
  Transfer Fcn : TransferFcn  Denominator=[L R + ron]
  Transfer Fcn1 : TransferFcn  Denominator=[L R + ron]
  Transfer Fcn2 : TransferFcn  Denominator=[L R + ron]
  Voltage Measurement{,1..7} (8 alike) : powerlib/Measurements/Voltage Measurement  PhasorSimulation=off  OutputType=Magnitude  PSBequivalent=0
  powergui : powerlib/powergui  Priority=1  SimulationMode=Continuous  SampleTime=50e-6  frequency=60  Iterations=50  frequencyindice=0  Pbase=100e6  ErrMax=1e-4  UnitsV=kV  UnitsW=MW  buscounter=0  FunctionMessages=off  echomessages=off  EnableUseOfTLC=off  CurrentSourceSwitches=off  DisableSnubberDevices=off  DisableRonSwitches=off  DisableVfSwitches=off  DisplayEquations=off  SolverType=Tustin/Backward Euler (TBE)  Interpol=off  ExternalGateDelay=off  methode=off  Ts=100  x0status=blocks  SPID=on  SwTol=0  HookPort=off  RestoreLinks=warning  ResistiveCurrentMeasurement=off  Frange=[0:2:500]  Ylog=off  Xlog=on  ShowGrid=off  save=off  variable=ZData  structure=0  ZoomFFT=off  StartTime=0.0  cycles=1  DisplayStyle=1  fundamental=60  FreqAxis=off  MaxFrequency=1000  frequencyindicesteady=1  RmsSteady=1  display=off
  i_out : Outport
  Us : Outport  Port=2
  VDC : Outport  Port=3
  IDC : Outport  Port=4
  PDC : Outport  Port=5
  wires:
  Manual Switch6/1 -> Multiply4/2
  Voltage Measurement1/1 -> Divide1/1, [V_cap_N]  "V_cap_N"
  Constant18/1 -> Switch11/1
  Voltage Measurement/1 -> Divide/2, [V_cap_P]  "V_cap_P"
  Divide/1 -> [I_DC_P], Controlled Current Source/1  "I_cap_in+"
  Constant7/1 -> Switch6/3
  Multiply4/1 -> Demux5/1
  [V_cap_P] -> Sum1/1
  Constant16/1 -> Switch9/1
  PID Controller/1 -> Subtract/1, Mux5/1
  Constant14/1 -> Switch7/3
  Constant17/1 -> Switch10/1
  Constant13/1 -> Manual Switch6/2
  Three-Phase V-I Measurement/2 -> i_out/1
  [V_cap_P] -> Subtract1/1
  Subtract/1 -> Mux5/2
  Mux5/1 -> Manual Switch6/1
  Sum1/1 -> PID Controller/1
  Divide3/1 -> Multiply15/2, Sum1/2
  Demux5/1 -> Divide/1
  Demux5/2 -> Divide1/2
  Constant15/1 -> Switch8/3
  [V_cap_N] -> Subtract1/2
  Three-Phase V-I Measurement/1 -> Us/1
  Constant8/1 -> Divide3/2
  Divide1/1 -> Controlled Current Source9/1, [I_DC_N]  "I_cap_in-"
  Demux6/1 -> Transfer Fcn1/1
  Demux6/2 -> Transfer Fcn/1
  Demux6/3 -> Transfer Fcn2/1
  modulation_in/1 -> Multiply15/1
  DC_POWER_IN/1 -> Multiply4/1
  [I_A_High] -> Controlled Current Source4/1
  [I_B_High] -> Controlled Current Source5/1
  [I_C_High] -> Controlled Current Source6/1
  [I_B_Low] -> Controlled Current Source2/1
  [I_C_Low] -> Controlled Current Source3/1
  [I_A_Low] -> Controlled Current Source1/1
  Voltage Measurement2/1 -> [U_A_High]
  Voltage Measurement3/1 -> [U_B_High]
  Voltage Measurement4/1 -> [U_C_High]
  Voltage Measurement5/1 -> [U_A_Low]
  Voltage Measurement6/1 -> [U_B_Low]
  Voltage Measurement7/1 -> [U_C_Low]
  [I_A_High] -> Multiply5/1
  [U_A_High] -> Multiply5/2
  [U_B_High] -> Multiply7/2
  [I_B_High] -> Multiply7/1
  [U_C_High] -> Multiply8/2
  [I_C_High] -> Multiply8/1
  Multiply5/1 -> Add/1
  Multiply7/1 -> Add/2
  Multiply8/1 -> Add/3
  Add/1 -> Divide2/1
  [V_cap_P] -> Divide2/2
  Divide2/1 -> Gain/1
  [U_A_Low] -> Multiply9/2
  Multiply11/1 -> Add1/3
  Add1/1 -> Divide4/1
  Multiply10/1 -> Add1/2
  [U_C_Low] -> Multiply11/2
  [I_C_Low] -> Multiply11/1
  [I_A_Low] -> Multiply9/1
  [U_B_Low] -> Multiply10/2
  [I_B_Low] -> Multiply10/1
  Multiply9/1 -> Add1/1
  [V_cap_N] -> Divide4/2
  Divide4/1 -> Gain1/1
  Gain1/1 -> Controlled Current Source8/1
  Gain/1 -> Controlled Current Source7/1
  Current Measurement/1 -> [I_cap_P]
  Current Measurement1/1 -> [I_cap_N]
  [I_cap_P] -> RMS/1  "I_cap_P"
  [I_cap_N] -> RMS1/1  "I_cap_N"
  RMS/1 -> ?  "I_cap_RMS_P"
  RMS1/1 -> ?  "I_cap_RMS_N"
  Step/1 -> Ideal Switch/1
  Switch8/1 -> [I_C_High]
  Switch7/1 -> [I_B_High]
  Switch6/1 -> [I_A_High]
  Switch11/1 -> [I_C_Low]
  Switch10/1 -> [I_B_Low]
  Switch9/1 -> [I_A_Low]
  Subtract1/1 -> Divide3/1
  Multiply15/1 -> Demux6/1
  Transfer Fcn1/1 -> Switch6/1, Switch6/2, Switch9/3, Switch9/2
  Transfer Fcn/1 -> Switch7/1, Switch7/2, Switch10/3, Switch10/2
  Transfer Fcn2/1 -> Switch11/3, Switch11/2, Switch8/1, Switch8/2
  Constant10/1 -> Subtract/2
  Subtract2/1 -> IDC/1
  [I_DC_P] -> Subtract2/1
  [I_DC_N] -> Subtract2/2
  [V_cap_P] -> Subtract3/1
  [V_cap_N] -> Subtract3/2
  Subtract3/1 -> VDC/1
  Subtract4/1 -> PDC/1
  [I_DC_P] -> Multiply/1
  [V_cap_P] -> Multiply/2
  [I_DC_N] -> Multiply1/1
  [V_cap_N] -> Multiply1/2
  Multiply/1 -> Subtract4/1
  Multiply1/1 -> Subtract4/2
  connections:
  Series RLC Branch2/LConn1 -- Voltage Measurement/LConn1 -- Controlled Current Source7/LConn1 -- Current Measurement/LConn1
  Controlled Current Source/LConn1 -- Controlled Current Source9/LConn1 -- Voltage Measurement/LConn2 -- Series RLC Branch/RConn1 -- Controlled Current Source7/RConn1 -- Ground1/LConn1 -- Controlled Current Source8/RConn1 -- Series RLC Branch1/LConn1 -- Voltage Measurement1/LConn2
  Controlled Current Source8/LConn1 -- Current Measurement1/LConn1 -- Series RLC Branch9/LConn1 -- Voltage Measurement1/LConn1
  Three-Phase Source/RConn3 -- Three-Phase Series RLC Branch/RConn3
  Controlled Current Source/RConn1 -- Series RLC Branch2/RConn1
  Ground2/LConn1 -- Three-Phase Source/LConn1
  Controlled Current Source1/RConn1 -- Voltage Measurement5/LConn2 -- Series RLC Branch3/LConn1 -- Three-Phase Series RLC Branch1/LConn1 -- Voltage Measurement2/LConn2 -- Series RLC Branch6/RConn1 -- Controlled Current Source4/RConn1
  Three-Phase Source/RConn2 -- Three-Phase Series RLC Branch/RConn2
  Controlled Current Source2/RConn1 -- Voltage Measurement6/LConn2 -- Series RLC Branch4/LConn1 -- Three-Phase Series RLC Branch1/LConn2 -- Voltage Measurement3/LConn2 -- Series RLC Branch7/RConn1 -- Controlled Current Source5/RConn1
  Three-Phase Source/RConn1 -- Three-Phase Series RLC Branch/RConn1
  Controlled Current Source3/RConn1 -- Voltage Measurement7/LConn2 -- Series RLC Branch5/LConn1 -- Voltage Measurement4/LConn2 -- Series RLC Branch8/RConn1 -- Controlled Current Source6/RConn1 -- Three-Phase Series RLC Branch1/LConn3
  Three-Phase Series RLC Branch/LConn1 -- Series RLC Branch10/LConn1 -- Three-Phase V-I Measurement/RConn1
  Three-Phase Series RLC Branch/LConn2 -- Three-Phase V-I Measurement/RConn2
  Three-Phase Series RLC Branch/LConn3 -- Three-Phase V-I Measurement/RConn3
  Series RLC Branch4/RConn1 -- Voltage Measurement6/LConn1 -- Ground6/LConn1 -- Controlled Current Source2/LConn1
  Controlled Current Source9/RConn1 -- Series RLC Branch9/RConn1
  Ideal Switch/RConn1 -- Series RLC Branch10/RConn1
  Series RLC Branch/LConn1 -- Current Measurement/RConn1
  Series RLC Branch1/RConn1 -- Current Measurement1/RConn1
  Ideal Switch/LConn1 -- Ground5/LConn1
  Series RLC Branch3/RConn1 -- Voltage Measurement5/LConn1 -- Ground4/LConn1 -- Controlled Current Source1/LConn1
  Controlled Current Source5/LConn1 -- Ground8/LConn1 -- Voltage Measurement3/LConn1 -- Series RLC Branch7/LConn1
  Series RLC Branch5/RConn1 -- Ground7/LConn1 -- Controlled Current Source3/LConn1 -- Voltage Measurement7/LConn1
  Ground3/LConn1 -- Controlled Current Source4/LConn1 -- Series RLC Branch6/LConn1 -- Voltage Measurement2/LConn1
  Voltage Measurement4/LConn1 -- Controlled Current Source6/LConn1 -- Series RLC Branch8/LConn1 -- Ground9/LConn1
  Three-Phase Series RLC Branch1/RConn1 -- Three-Phase V-I Measurement/LConn1
  Three-Phase Series RLC Branch1/RConn2 -- Three-Phase V-I Measurement/LConn2
  Three-Phase Series RLC Branch1/RConn3 -- Three-Phase V-I Measurement/LConn3

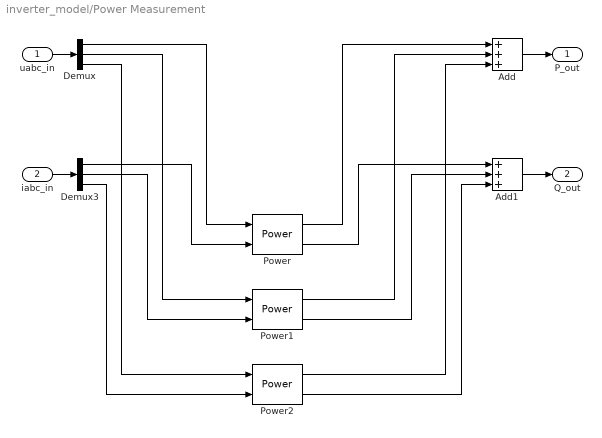
== system inverter_model/Power Measurement ==
  uabc_in : Inport
  iabc_in : Inport  Port=2
  Add : Sum  Inputs=3
  Add1 : Sum  Inputs=3
  Demux : Demux  Outputs=3
  Demux3 : Demux  Outputs=3
  Power : powerlib_meascontrol/Measurements/Power  Freq=50  Vinit=[1, 0]  Iinit=[1, 0]  Ts=0
      settings: SourceProductName=Simscape Electrical
  Power1 : powerlib_meascontrol/Measurements/Power  Freq=50  Vinit=[1, 0]  Iinit=[1, 0]  Ts=0
      settings: SourceProductName=Simscape Electrical
  Power2 : powerlib_meascontrol/Measurements/Power  Freq=50  Vinit=[1, 0]  Iinit=[1, 0]  Ts=0
      settings: SourceProductName=Simscape Electrical
  P_out : Outport
  Q_out : Outport  Port=2
  wires:
  Demux/2 -> Power1/1
  Power/2 -> Add1/1
  Demux3/2 -> Power1/2
  Demux/3 -> Power2/1
  Demux/1 -> Power/1
  Demux3/3 -> Power2/2
  Power2/1 -> Add/3
  Power1/1 -> Add/2
  Power1/2 -> Add1/2
  Demux3/1 -> Power/2
  Power/1 -> Add/1
  Power2/2 -> Add1/3
  iabc_in/1 -> Demux3/1
  uabc_in/1 -> Demux/1
  Add/1 -> P_out/1
  Add1/1 -> Q_out/1

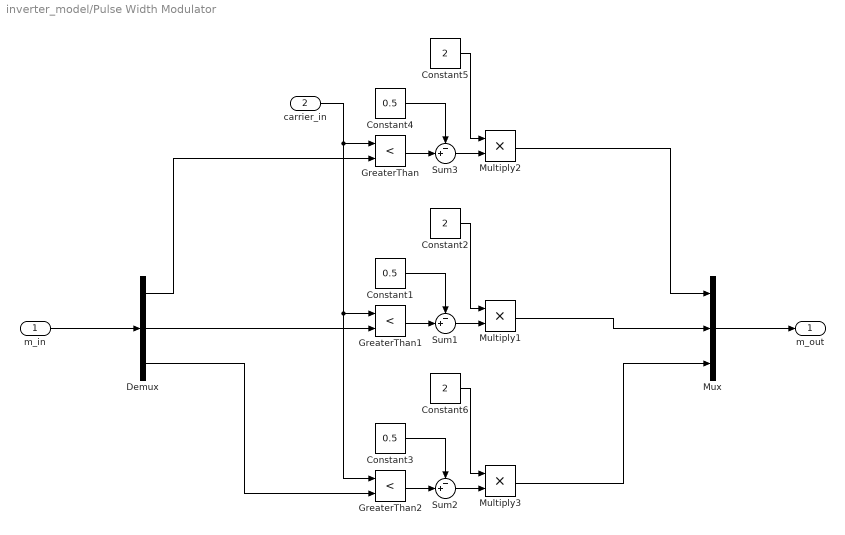
== system inverter_model/Pulse Width Modulator ==
  m_in : Inport
  carrier_in : Inport  Port=2
  Constant1 : Constant  Value=0.5
  Constant2 : Constant  Value=2
  Constant3 : Constant  Value=0.5
  Constant4 : Constant  Value=0.5
  Constant5 : Constant  Value=2
  Constant6 : Constant  Value=2
  Demux : Demux  Outputs=3
  GreaterThan : RelationalOperator  Operator=<  OutDataTypeStr=boolean  RndMeth=Simplest
  GreaterThan1 : RelationalOperator  Operator=<  OutDataTypeStr=boolean  RndMeth=Simplest
  GreaterThan2 : RelationalOperator  Operator=<  OutDataTypeStr=boolean  RndMeth=Simplest
  Multiply1 : Product
  Multiply2 : Product
  Multiply3 : Product
  Mux : Mux  Inputs=3
  Sum1 : Sum  Inputs=-+|
  Sum2 : Sum  Inputs=-+|
  Sum3 : Sum  Inputs=-+|
  "m_out " : Outport
  wires:
  Multiply2/1 -> Mux/1
  GreaterThan/1 -> Sum3/2
  Constant4/1 -> Sum3/1
  Constant5/1 -> Multiply2/1
  Sum3/1 -> Multiply2/2
  m_in/1 -> Demux/1
  Mux/1 -> "m_out "/1
  carrier_in/1 -> GreaterThan2/1, GreaterThan1/1, GreaterThan/1
  Demux/1 -> GreaterThan/2
  Constant2/1 -> Multiply1/1
  Constant1/1 -> Sum1/1
  GreaterThan1/1 -> Sum1/2
  Sum1/1 -> Multiply1/2
  Demux/2 -> GreaterThan1/2
  Multiply1/1 -> Mux/2
  Constant6/1 -> Multiply3/1
  Constant3/1 -> Sum2/1
  GreaterThan2/1 -> Sum2/2
  Sum2/1 -> Multiply3/2
  Demux/3 -> GreaterThan2/2
  Multiply3/1 -> Mux/3
